simulink model "test_NetworkInterface_UDP_InputOutput"  (R2016b)
settings: Solver=FixedStepDiscrete  StartTime=0.0  StopTime=inf  FixedStep=0.05  RelTol=1e-3
libraries: simulink x1, LIB_NetwokInterface x1
settings Model: SimulationMode=external  ExtModeTrigDuration=10000  Creator=constantin  LastModifiedBy=valtin
settings DataIOCC: LimitDataPoints=on  SaveFormat=Array
settings OptimizationCC: ExpressionDepthLimit=2147483647  LifeSpan=1
settings DebuggingCC: UnderspecifiedInitializationDetection=Classic  MergeDetectMultiDrivingBlocksExec=none  SolverPrmCheckMsg=warning  StateNameClashWarn=warning  SFUnexpectedBacktrackingDiag=warning  SFNoUnconditionalDefaultTransitionDiag=warning  SFExecutionAtInitializationDiag=none
settings HardwareCC: ProdBitPerPointer=32  ProdBitPerSizeT=32  ProdBitPerPtrDiffT=32  ProdLargestAtomicFloat=None  ProdIntDivRoundTo=Undefined  ProdEndianess=Unspecified  ProdWordSize=32  ProdHWDeviceType=32-bit Generic
settings ModelReferenceCC: PropagateSignalLabelsOutOfModel=off
settings SFSimCC: SimParseCustomCode=off
settings RTWCC: SystemTargetFile=ert_linux.tlc  MakeCommand=make_rtw OPTS=-DWITH_HW OPTIMIZATION_FLAGS=-O3  TemplateMakefile=ert_linux.tmf  Description=Linux Embedded Coder  TargetLang=C++
settings CodeAppCC: IgnoreCustomStorageClasses=off  CustomSymbolStrType=$N$R$M  InternalIdentifier=Classic
settings STFCustomTargetCC: ModelReferenceCompliant=off  GeneratePreprocessorConditionals=Disable all  CombineOutputUpdateFcns=on  ERTCustomFileBanners=on  SupportComplex=off  RemoveResetFunc=on  SupportVariableSizeSignals=on  MATLABClassNameForMDSCustomization=Simulink.SoftwareTarget.ERTCustomization  GRTInterface=off  SystemTargetFile=ert_linux.tlc
settings ERTTargetCC: ModelReferenceCompliant=off  ParMdlRefBuildCompliant=off  CompOptLevelCompliant=off  ConcurrentExecutionCompliant=off  GeneratePreprocessorConditionals=Disable all  ERTFirstTimeCompliant=off  SupportComplex=off  SupportContinuousTime=on  SupportNonInlinedSFcns=on  SupportVariableSizeSignals=on  ModelStepFunctionPrototypeControlCompliant=off  CPPClassGenCompliant=off  UseToolchainInfoCompliant=off  ExtMode=on  MultiInstanceErrorCode=None  ERTCustomFileTemplate=ert_linux_file_process.tlc  ConvertIfToSwitch=off  SuppressUnreachableDefaultCases=off
settings ConfigComp: CovMetricSettings=dw  CovHtmlReporting=on  CovSaveCumulativeToWorkspaceVar=on  CovSaveSingleToWorkspaceVar=on  CovExternalEMLEnable=off  CovSFcnEnable=off
settings ConfigurationSet: Description=SimMechanics 2G

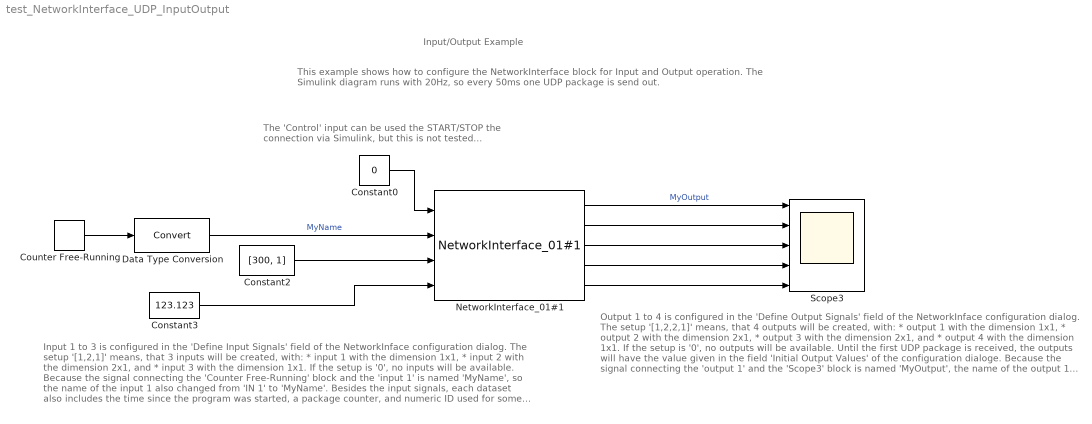
== system test_NetworkInterface_UDP_InputOutput ==
  note: Input/Output Example
  note: This example shows how to configure the NetworkInterface block for Input and Output operation.
      | The Simulink diagram runs with 20Hz, so every 50ms one UDP package is send out.
  note: The 'Control' input can be used the START/STOP
      | the connection via Simulink, but this is not tested...
  note: Input 1 to 3 is configured in the 'Define Input Signals' field of the NetworkInface configuration dialog.
      | The setup '[1,2,1]' means, that 3 inputs will be created, with:
      |  * input 1 with the dimension 1x1,
      |  * input 2 with the dimension 2x1, and
      |  * input 3 with the dimension 1x1.
      | If the setup is '0', no inputs will be available.
      |
      | Because the signal connecting the 'Counter Free-Running' block and the 'input 1' is named 'MyName',
      | so the name of the input 1 also changed from 'IN 1' to 'MyName'.
      |
      | Besides the input signals, each dataset also includes the time since the program was started,
      | a package counter, and numeric ID used for some rudimentary check's.
  note: Output 1 to 4 is configured in the 'Define Output Signals' field of the NetworkInface configuration dialog.
      | The setup '[1,2,2,1]' means, that 4 outputs will be created, with:
      |  * output 1 with the dimension 1x1,
      |  * output 2 with the dimension 2x1,
      |  * output 3 with the dimension 2x1, and
      |  * output 4 with the dimension 1x1.
      | If the setup is '0', no outputs will be available.
      |
      | Until the first UDP package is received, the outputs will have the value given in the field
      | 'Initial Output Values' of the configuration dialoge.
      |
      | Because the signal connecting the 'output 1' and the 'Scope3' block is named 'MyOutput',
      | the name of the output 1 also changed from 'OUT 1' to 'MyOutput'.
      |
      | The 'MsgCounter' output counts the number of received dataset's and can be used to detect missing
      | packages or a lost connection. However, please consider that there is NO synchronisation and NO
      | garantied timing for the UDP connection.
  Constant0 : Constant  Value=0  OutDataTypeStr=double  SampleTime=-1
  Constant2 : Constant  Value=[300, 1]  OutDataTypeStr=double  SampleTime=-1
  Constant3 : Constant  Value=123.123  OutDataTypeStr=double  SampleTime=-1
  Counter Free-Running : simulink/Sources/Counter Free-Running  NumBits=16  tsamp=-1
  Data Type Conversion : DataTypeConversion
  NetworkInterface_01#1 : LIB_NetwokInterface/NetworkInterface_01#1  inputs=[1,2,1]  outputs=[1,2,2,1]  initialOutputValues=1  SampleTime=-1  useUDP=on  startConnection=on  localPort=20000  remoteIP='127.0.0.1'  remotePort=20001
  Scope3 : Scope  NumInputPorts=5
  wires:
  NetworkInterface_01#1/1 -> Scope3/1  "MyOutput"
  NetworkInterface_01#1/2 -> Scope3/2
  Constant2/1 -> NetworkInterface_01#1/3
  Constant3/1 -> NetworkInterface_01#1/4
  Constant0/1 -> NetworkInterface_01#1/1
  NetworkInterface_01#1/3 -> Scope3/3
  NetworkInterface_01#1/4 -> Scope3/4
  NetworkInterface_01#1/5 -> Scope3/5
  Counter Free-Running/1 -> Data Type Conversion/1
  Data Type Conversion/1 -> NetworkInterface_01#1/2  "MyName"
